simulink model "Lab5"  (R2018b)
settings: Solver=VariableStepAuto  StartTime=0.0  StopTime=0.7  RelTol=1e-3
values from neighbouring files (symbols this model uses):
  kpp = w_cp    (= 60)    [Lab5.m]
  kpv1 = w_cv/mu1    (= 0.09888)    [Lab5.m]
  kpv2 = w_cv/mu2    (= 0.114)    [Lab5.m]
  kpv3 = w_cv/mu3    (= 0.0408)    [Lab5.m]
  kpv4 = w_cv/mu4    (= 0.004056)    [Lab5.m]
  kpv5 = w_cv/mu5    (= 0.0031338)    [Lab5.m]
  kpv6 = w_cv/mu6    (= 0.003006)    [Lab5.m]
  n1 = 100    [Lab5.m]
  n2 = n1    (= 100)    [Lab5.m]
  n3 = n1    (= 100)    [Lab5.m]
  n4 = n1    (= 100)    [Lab5.m]
  n5 = n1    (= 100)    [Lab5.m]
  n6 = n1    (= 100)    [Lab5.m]
  t0 = 0.1    [Lab5.m]
  t_acc = (t_tot*x_dot_max-x_displacement)/x_dot_max    (= 0.1)    [Lab5.m]
  t_tot = 0.5    [Lab5.m]
  Tiv = 1/(0.2*w_cv)    (= 0.00833333333333)    [Lab5.m]
  x0 = 0.2    [Lab5.m]
  x_dotdot = x_dot_max/t_acc    (= 10)    [Lab5.m]
libraries: simulink x6, roblocks x1
settings Model: Creator=costanza  LastModifiedBy=costanza

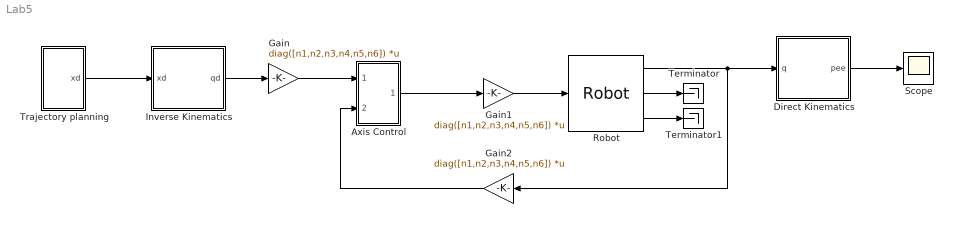
== system Lab5 ==
  "Axis Control " : Subsystem
  Direct Kinematics : Subsystem
  Gain : Gain  Gain=diag([n1,n2,n3,n4,n5,n6])  Multiplication=Matrix(K*u)
  Gain1 : Gain  Gain=diag([n1,n2,n3,n4,n5,n6])  Multiplication=Matrix(K*u)
  Gain2 : Gain  Gain=diag([n1,n2,n3,n4,n5,n6])  Multiplication=Matrix(K*u)
  Inverse Kinematics : Subsystem
  Robot : roblocks/Arm/Robot  robot=UR5  q0=q_init'
  Scope : Scope
  Terminator : Terminator
  Terminator1 : Terminator
  "Trajectory planning " : Subsystem
  wires:
  Gain/1 -> "Axis Control "/1(qmd)
  "Axis Control "/1("taum ") -> Gain1/1
  Gain1/1 -> Robot/1
  Robot/2 -> Terminator/1
  Robot/3 -> Terminator1/1
  Gain2/1 -> "Axis Control "/2(qm)
  Robot/1 -> Direct Kinematics/1("q "), Gain2/1
  Direct Kinematics/1(pee) -> Scope/1
  "Trajectory planning "/1(xd) -> Inverse Kinematics/1(xd)
  Inverse Kinematics/1(qd) -> Gain/1

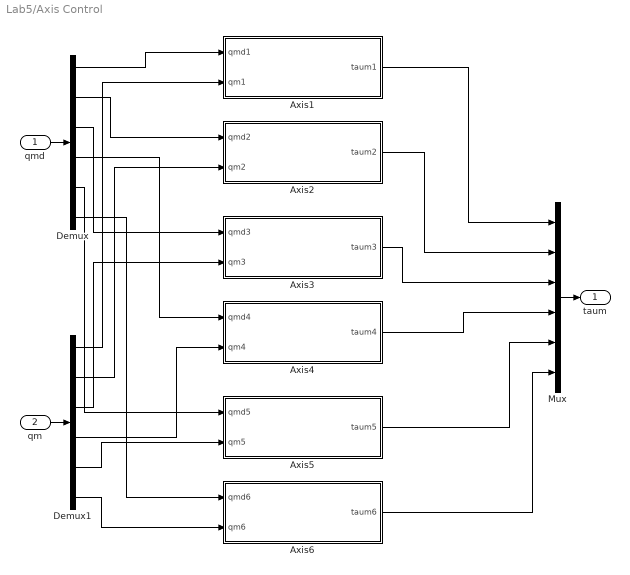
== system Lab5/Axis Control  ==
  qmd : Inport
  qm : Inport  Port=2
  "Axis1 " : Subsystem
  "Axis2 " : Subsystem
  "Axis3 " : Subsystem
  "Axis4 " : Subsystem
  "Axis5 " : Subsystem
  "Axis6 " : Subsystem
  Demux : Demux  Outputs=6
  Demux1 : Demux  Outputs=6
  Mux : Mux  Inputs=6
  "taum " : Outport
  wires:
  "Axis5 "/1(taum5) -> Mux/5
  Demux1/1 -> "Axis1 "/2(qm1)
  "Axis2 "/1(taum2) -> Mux/2
  Demux1/3 -> "Axis3 "/2(qm3)
  Demux/1 -> "Axis1 "/1(qmd1)
  "Axis4 "/1(taum4) -> Mux/4
  "Axis3 "/1(taum3) -> Mux/3
  "Axis6 "/1("taum6 ") -> Mux/6
  "Axis1 "/1(taum1) -> Mux/1
  Mux/1 -> "taum "/1
  Demux/2 -> "Axis2 "/1(qmd2)
  Demux/4 -> "Axis4 "/1(qmd4)
  Demux/3 -> "Axis3 "/1(qmd3)
  Demux/6 -> "Axis6 "/1(qmd6)
  Demux/5 -> "Axis5 "/1(qmd5)
  Demux1/4 -> "Axis4 "/2(qm4)
  Demux1/6 -> "Axis6 "/2(qm6)
  Demux1/5 -> "Axis5 "/2(qm5)
  Demux1/2 -> "Axis2 "/2(qm2)
  qm/1 -> Demux1/1
  qmd/1 -> Demux/1

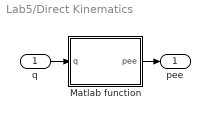
== system Lab5/Direct Kinematics ==
  "q " : Inport
  "Matlab function " : MATLAB Function  TreatAsAtomicUnit=on
  pee : Outport
  wires:
  "q "/1 -> "Matlab function "/1(q)
  "Matlab function "/1(pee) -> pee/1

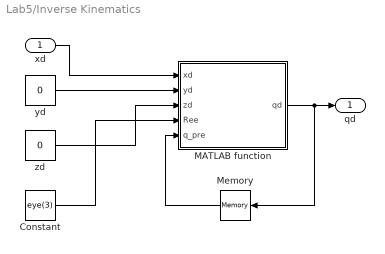
== system Lab5/Inverse Kinematics ==
  xd : Inport
  Constant : Constant  Value=eye(3)  VectorParams1D=off
  "MATLAB function " : MATLAB Function  TreatAsAtomicUnit=on
  Memory : Memory  InitialCondition=q_init'
  yd : Constant  Value=0
  "zd " : Constant  Value=0
  qd : Outport
  wires:
  xd/1 -> "MATLAB function "/1(xd)
  "MATLAB function "/1(qd) -> Memory/1, qd/1
  yd/1 -> "MATLAB function "/2(yd)
  "zd "/1 -> "MATLAB function "/3(zd)
  Constant/1 -> "MATLAB function "/4(Ree)
  Memory/1 -> "MATLAB function "/5(q_pre)

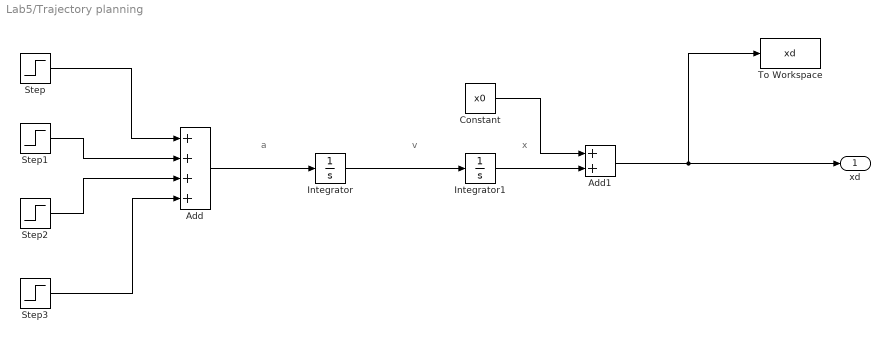
== system Lab5/Trajectory planning  ==
  note: a
  note: v
  note: x
  Add : Sum  Inputs=++++
  Add1 : Sum
  Constant : Constant  Value=x0
  Integrator : Integrator
  Integrator1 : Integrator
  Step : Step  Time=t0  After=x_dotdot  SampleTime=0
  Step1 : Step  Time=t0+t_acc  After=-x_dotdot  SampleTime=0
  Step2 : Step  Time=t0+t_tot-t_acc  After=-x_dotdot  SampleTime=0
  Step3 : Step  Time=t0+t_tot  After=x_dotdot  SampleTime=0
  To Workspace : ToWorkspace  VariableName=xd  SampleTime=-1
  xd : Outport
  wires:
  Step2/1 -> Add/3
  Step/1 -> Add/1
  Add/1 -> Integrator/1
  Step3/1 -> Add/4
  Step1/1 -> Add/2
  Integrator/1 -> Integrator1/1
  Add1/1 -> xd/1, To Workspace/1
  Constant/1 -> Add1/1
  Integrator1/1 -> Add1/2

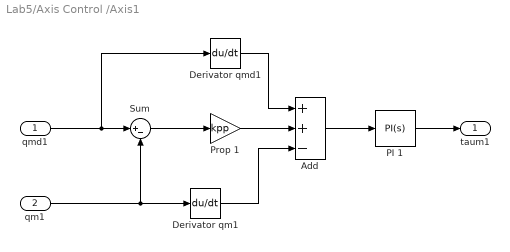
== system Lab5/Axis Control /Axis1  ==
  qmd1 : Inport
  qm1 : Inport  Port=2
  Add : Sum  Inputs=++-
  Derivator qm1 : Derivative  CoefficientInTFapproximation=1/260
  "Derivator qmd1 " : Derivative  CoefficientInTFapproximation=1/260
  PI 1 : simulink/Continuous/PID Controller  Controller=PI  Form=Parallel  TimeDomain=Continuous-time  SampleTime=-1  IntegratorMethod=Forward Euler  FilterMethod=Forward Euler  ControllerParametersSource=internal  P=kpv1  I=kpv1/Tiv  D=0  UseFilter=on  N=100  TunerSelectOption=Transfer Function Based (PID Tuner App)  InitialConditionSource=internal  InitialConditionForIntegrator=0  InitialConditionForFilter=0  DifferentiatorICPrevScaledInput=0  ExternalReset=none  TrackingMode=off  Kt=1  LimitOutput=off  UpperSaturationLimit=inf  LowerSaturationLimit=-inf  LinearizeAsGain=on  AntiWindupMode=none  Kb=1  POutMin=[]  POutMax=[]  IOutMin=[]  IOutMax=[]  DOutMin=[]  DOutMax=[]  NOutMin=[]  NOutMax=[]  SumOutMin=[]  SumOutMax=[]  SaturationOutMin=[]  SaturationOutMax=[]  PParamMin=[]  PParamMax=[]  IParamMin=[]  IParamMax=[]  DParamMin=[]  DParamMax=[]  NParamMin=[]  NParamMax=[]  KbParamMin=[]  KbParamMax=[]  KtParamMin=[]  KtParamMax=[]  KbOutMin=[]  KbOutMax=[]  KtOutMin=[]  KtOutMax=[]  IntegratorOutMin=[]  IntegratorOutMax=[]  FilterOutMin=[]  FilterOutMax=[]  SumI1OutMin=[]  SumI1OutMax=[]  SumI2OutMin=[]  SumI2OutMax=[]  SumI3OutMin=[]  SumI3OutMax=[]  SumI4OutMin=[]  SumI4OutMax=[]  SumDOutMin=[]  SumDOutMax=[]  DifferentiatorOutMin=[]  DifferentiatorOutMax=[]  FilterDiffOutCoefMin=[]  FilterDiffOutCoefMax=[]  ReciprocalOutMin=[]  ReciprocalOutMax=[]  SumDenOutMin=[]  SumDenOutMax=[]  SumNumOutMin=[]  SumNumOutMax=[]  DivideOutMin=[]  DivideOutMax=[]  IntegratorContinuousStateAttributes=''  IntegratorStateMustResolveToSignalObject=off  IntegratorRTWStateStorageClass=Auto  FilterContinuousStateAttributes=''  FilterStateMustResolveToSignalObject=off  FilterRTWStateStorageClass=Auto  ParallelPVariant=InternalParameters  IdealPVariant=Disabled  IVariant=InternalParameters  DVariant=Disabled  IntegratorVariant=Continuous  SatVariant=Disabled  AWVariant=Passthrough  PCopyVariant=Disabled  TRVariant=Disabled  FdbkBlocksVariant=Forward  IdealPFdbkVariant=Disabled  SatFdbkVariant=Disabled  DerivativeFilterVariant=Disabled  NVariant=Disabled  NCopyVariant=Disabled_SignalSpec  FilterICVariant=Disabled  IntegratorICVariant=InternalICs  ExternalResetVariant=Disabled  TRSumVariant=Passthrough  SumFdbkVariant=Disabled  SumVariant=Sum_PI
  Prop 1 : Gain  Gain=kpp
  Sum : Sum  Inputs=|+-
  taum1 : Outport
  wires:
  "Derivator qmd1 "/1 -> Add/1
  Derivator qm1/1 -> Add/3
  Sum/1 -> Prop 1/1
  qm1/1 -> Derivator qm1/1, Sum/2
  Prop 1/1 -> Add/2
  Add/1 -> PI 1/1
  qmd1/1 -> "Derivator qmd1 "/1, Sum/1
  PI 1/1 -> taum1/1

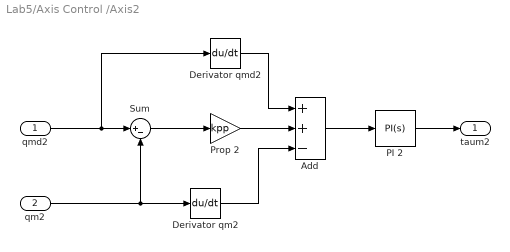
== system Lab5/Axis Control /Axis2  ==
  qmd2 : Inport
  qm2 : Inport  Port=2
  Add : Sum  Inputs=++-
  Derivator qm2 : Derivative  CoefficientInTFapproximation=1/260
  Derivator qmd2 : Derivative  CoefficientInTFapproximation=1/260
  PI 2 : simulink/Continuous/PID Controller  Controller=PI  Form=Parallel  TimeDomain=Continuous-time  SampleTime=-1  IntegratorMethod=Forward Euler  FilterMethod=Forward Euler  ControllerParametersSource=internal  P=kpv2  I=kpv2/Tiv  D=0  UseFilter=on  N=100  TunerSelectOption=Transfer Function Based (PID Tuner App)  InitialConditionSource=internal  InitialConditionForIntegrator=0  InitialConditionForFilter=0  DifferentiatorICPrevScaledInput=0  ExternalReset=none  TrackingMode=off  Kt=1  LimitOutput=off  UpperSaturationLimit=inf  LowerSaturationLimit=-inf  LinearizeAsGain=on  AntiWindupMode=none  Kb=1  POutMin=[]  POutMax=[]  IOutMin=[]  IOutMax=[]  DOutMin=[]  DOutMax=[]  NOutMin=[]  NOutMax=[]  SumOutMin=[]  SumOutMax=[]  SaturationOutMin=[]  SaturationOutMax=[]  PParamMin=[]  PParamMax=[]  IParamMin=[]  IParamMax=[]  DParamMin=[]  DParamMax=[]  NParamMin=[]  NParamMax=[]  KbParamMin=[]  KbParamMax=[]  KtParamMin=[]  KtParamMax=[]  KbOutMin=[]  KbOutMax=[]  KtOutMin=[]  KtOutMax=[]  IntegratorOutMin=[]  IntegratorOutMax=[]  FilterOutMin=[]  FilterOutMax=[]  SumI1OutMin=[]  SumI1OutMax=[]  SumI2OutMin=[]  SumI2OutMax=[]  SumI3OutMin=[]  SumI3OutMax=[]  SumI4OutMin=[]  SumI4OutMax=[]  SumDOutMin=[]  SumDOutMax=[]  DifferentiatorOutMin=[]  DifferentiatorOutMax=[]  FilterDiffOutCoefMin=[]  FilterDiffOutCoefMax=[]  ReciprocalOutMin=[]  ReciprocalOutMax=[]  SumDenOutMin=[]  SumDenOutMax=[]  SumNumOutMin=[]  SumNumOutMax=[]  DivideOutMin=[]  DivideOutMax=[]  IntegratorContinuousStateAttributes=''  IntegratorStateMustResolveToSignalObject=off  IntegratorRTWStateStorageClass=Auto  FilterContinuousStateAttributes=''  FilterStateMustResolveToSignalObject=off  FilterRTWStateStorageClass=Auto  ParallelPVariant=InternalParameters  IdealPVariant=Disabled  IVariant=InternalParameters  DVariant=Disabled  IntegratorVariant=Continuous  SatVariant=Disabled  AWVariant=Passthrough  PCopyVariant=Disabled  TRVariant=Disabled  FdbkBlocksVariant=Forward  IdealPFdbkVariant=Disabled  SatFdbkVariant=Disabled  DerivativeFilterVariant=Disabled  NVariant=Disabled  NCopyVariant=Disabled_SignalSpec  FilterICVariant=Disabled  IntegratorICVariant=InternalICs  ExternalResetVariant=Disabled  TRSumVariant=Passthrough  SumFdbkVariant=Disabled  SumVariant=Sum_PI
  Prop 2 : Gain  Gain=kpp
  Sum : Sum  Inputs=|+-
  taum2 : Outport
  wires:
  Derivator qmd2/1 -> Add/1
  Derivator qm2/1 -> Add/3
  Sum/1 -> Prop 2/1
  qm2/1 -> Derivator qm2/1, Sum/2
  Prop 2/1 -> Add/2
  Add/1 -> PI 2/1
  qmd2/1 -> Derivator qmd2/1, Sum/1
  PI 2/1 -> taum2/1

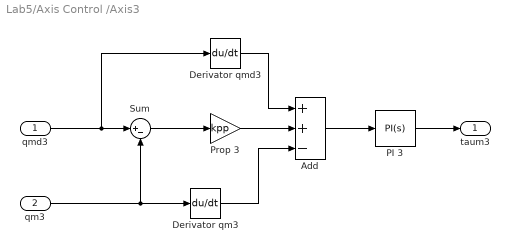
== system Lab5/Axis Control /Axis3  ==
  qmd3 : Inport
  qm3 : Inport  Port=2
  Add : Sum  Inputs=++-
  Derivator qm3 : Derivative  CoefficientInTFapproximation=1/260
  Derivator qmd3 : Derivative  CoefficientInTFapproximation=1/260
  PI 3 : simulink/Continuous/PID Controller  Controller=PI  Form=Parallel  TimeDomain=Continuous-time  SampleTime=-1  IntegratorMethod=Forward Euler  FilterMethod=Forward Euler  ControllerParametersSource=internal  P=kpv3  I=kpv3/Tiv  D=0  UseFilter=on  N=100  TunerSelectOption=Transfer Function Based (PID Tuner App)  InitialConditionSource=internal  InitialConditionForIntegrator=0  InitialConditionForFilter=0  DifferentiatorICPrevScaledInput=0  ExternalReset=none  TrackingMode=off  Kt=1  LimitOutput=off  UpperSaturationLimit=inf  LowerSaturationLimit=-inf  LinearizeAsGain=on  AntiWindupMode=none  Kb=1  POutMin=[]  POutMax=[]  IOutMin=[]  IOutMax=[]  DOutMin=[]  DOutMax=[]  NOutMin=[]  NOutMax=[]  SumOutMin=[]  SumOutMax=[]  SaturationOutMin=[]  SaturationOutMax=[]  PParamMin=[]  PParamMax=[]  IParamMin=[]  IParamMax=[]  DParamMin=[]  DParamMax=[]  NParamMin=[]  NParamMax=[]  KbParamMin=[]  KbParamMax=[]  KtParamMin=[]  KtParamMax=[]  KbOutMin=[]  KbOutMax=[]  KtOutMin=[]  KtOutMax=[]  IntegratorOutMin=[]  IntegratorOutMax=[]  FilterOutMin=[]  FilterOutMax=[]  SumI1OutMin=[]  SumI1OutMax=[]  SumI2OutMin=[]  SumI2OutMax=[]  SumI3OutMin=[]  SumI3OutMax=[]  SumI4OutMin=[]  SumI4OutMax=[]  SumDOutMin=[]  SumDOutMax=[]  DifferentiatorOutMin=[]  DifferentiatorOutMax=[]  FilterDiffOutCoefMin=[]  FilterDiffOutCoefMax=[]  ReciprocalOutMin=[]  ReciprocalOutMax=[]  SumDenOutMin=[]  SumDenOutMax=[]  SumNumOutMin=[]  SumNumOutMax=[]  DivideOutMin=[]  DivideOutMax=[]  IntegratorContinuousStateAttributes=''  IntegratorStateMustResolveToSignalObject=off  IntegratorRTWStateStorageClass=Auto  FilterContinuousStateAttributes=''  FilterStateMustResolveToSignalObject=off  FilterRTWStateStorageClass=Auto  ParallelPVariant=InternalParameters  IdealPVariant=Disabled  IVariant=InternalParameters  DVariant=Disabled  IntegratorVariant=Continuous  SatVariant=Disabled  AWVariant=Passthrough  PCopyVariant=Disabled  TRVariant=Disabled  FdbkBlocksVariant=Forward  IdealPFdbkVariant=Disabled  SatFdbkVariant=Disabled  DerivativeFilterVariant=Disabled  NVariant=Disabled  NCopyVariant=Disabled_SignalSpec  FilterICVariant=Disabled  IntegratorICVariant=InternalICs  ExternalResetVariant=Disabled  TRSumVariant=Passthrough  SumFdbkVariant=Disabled  SumVariant=Sum_PI
  Prop 3 : Gain  Gain=kpp
  Sum : Sum  Inputs=|+-
  taum3 : Outport
  wires:
  Derivator qmd3/1 -> Add/1
  Derivator qm3/1 -> Add/3
  Sum/1 -> Prop 3/1
  qm3/1 -> Derivator qm3/1, Sum/2
  Prop 3/1 -> Add/2
  Add/1 -> PI 3/1
  qmd3/1 -> Derivator qmd3/1, Sum/1
  PI 3/1 -> taum3/1

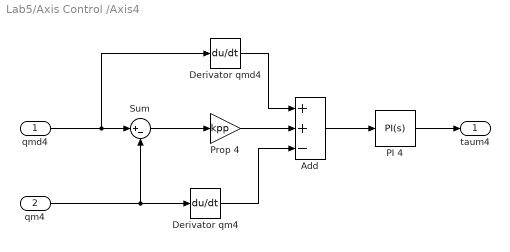
== system Lab5/Axis Control /Axis4  ==
  qmd4 : Inport
  qm4 : Inport  Port=2
  Add : Sum  Inputs=++-
  Derivator qm4 : Derivative  CoefficientInTFapproximation=1/700
  Derivator qmd4 : Derivative  CoefficientInTFapproximation=1/700
  PI 4 : simulink/Continuous/PID Controller  Controller=PI  Form=Parallel  TimeDomain=Continuous-time  SampleTime=-1  IntegratorMethod=Forward Euler  FilterMethod=Forward Euler  ControllerParametersSource=internal  P=kpv4  I=kpv4/Tiv  D=0  UseFilter=on  N=100  TunerSelectOption=Transfer Function Based (PID Tuner App)  InitialConditionSource=internal  InitialConditionForIntegrator=0  InitialConditionForFilter=0  DifferentiatorICPrevScaledInput=0  ExternalReset=none  TrackingMode=off  Kt=1  LimitOutput=off  UpperSaturationLimit=inf  LowerSaturationLimit=-inf  LinearizeAsGain=on  AntiWindupMode=none  Kb=1  POutMin=[]  POutMax=[]  IOutMin=[]  IOutMax=[]  DOutMin=[]  DOutMax=[]  NOutMin=[]  NOutMax=[]  SumOutMin=[]  SumOutMax=[]  SaturationOutMin=[]  SaturationOutMax=[]  PParamMin=[]  PParamMax=[]  IParamMin=[]  IParamMax=[]  DParamMin=[]  DParamMax=[]  NParamMin=[]  NParamMax=[]  KbParamMin=[]  KbParamMax=[]  KtParamMin=[]  KtParamMax=[]  KbOutMin=[]  KbOutMax=[]  KtOutMin=[]  KtOutMax=[]  IntegratorOutMin=[]  IntegratorOutMax=[]  FilterOutMin=[]  FilterOutMax=[]  SumI1OutMin=[]  SumI1OutMax=[]  SumI2OutMin=[]  SumI2OutMax=[]  SumI3OutMin=[]  SumI3OutMax=[]  SumI4OutMin=[]  SumI4OutMax=[]  SumDOutMin=[]  SumDOutMax=[]  DifferentiatorOutMin=[]  DifferentiatorOutMax=[]  FilterDiffOutCoefMin=[]  FilterDiffOutCoefMax=[]  ReciprocalOutMin=[]  ReciprocalOutMax=[]  SumDenOutMin=[]  SumDenOutMax=[]  SumNumOutMin=[]  SumNumOutMax=[]  DivideOutMin=[]  DivideOutMax=[]  IntegratorContinuousStateAttributes=''  IntegratorStateMustResolveToSignalObject=off  IntegratorRTWStateStorageClass=Auto  FilterContinuousStateAttributes=''  FilterStateMustResolveToSignalObject=off  FilterRTWStateStorageClass=Auto  ParallelPVariant=InternalParameters  IdealPVariant=Disabled  IVariant=InternalParameters  DVariant=Disabled  IntegratorVariant=Continuous  SatVariant=Disabled  AWVariant=Passthrough  PCopyVariant=Disabled  TRVariant=Disabled  FdbkBlocksVariant=Forward  IdealPFdbkVariant=Disabled  SatFdbkVariant=Disabled  DerivativeFilterVariant=Disabled  NVariant=Disabled  NCopyVariant=Disabled_SignalSpec  FilterICVariant=Disabled  IntegratorICVariant=InternalICs  ExternalResetVariant=Disabled  TRSumVariant=Passthrough  SumFdbkVariant=Disabled  SumVariant=Sum_PI
  Prop 4 : Gain  Gain=kpp
  Sum : Sum  Inputs=|+-
  taum4 : Outport
  wires:
  Derivator qmd4/1 -> Add/1
  Derivator qm4/1 -> Add/3
  Sum/1 -> Prop 4/1
  qm4/1 -> Derivator qm4/1, Sum/2
  Prop 4/1 -> Add/2
  Add/1 -> PI 4/1
  qmd4/1 -> Derivator qmd4/1, Sum/1
  PI 4/1 -> taum4/1

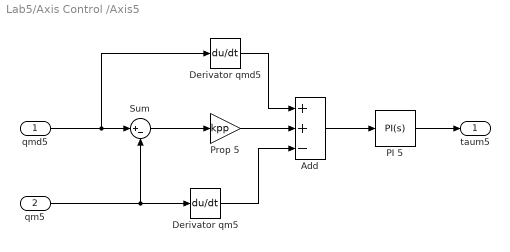
== system Lab5/Axis Control /Axis5  ==
  qmd5 : Inport
  qm5 : Inport  Port=2
  Add : Sum  Inputs=++-
  Derivator qm5 : Derivative  CoefficientInTFapproximation=1/700
  Derivator qmd5 : Derivative  CoefficientInTFapproximation=1/700
  PI 5 : simulink/Continuous/PID Controller  Controller=PI  Form=Parallel  TimeDomain=Continuous-time  SampleTime=-1  IntegratorMethod=Forward Euler  FilterMethod=Forward Euler  ControllerParametersSource=internal  P=kpv5  I=kpv5/Tiv  D=0  UseFilter=on  N=100  TunerSelectOption=Transfer Function Based (PID Tuner App)  InitialConditionSource=internal  InitialConditionForIntegrator=0  InitialConditionForFilter=0  DifferentiatorICPrevScaledInput=0  ExternalReset=none  TrackingMode=off  Kt=1  LimitOutput=off  UpperSaturationLimit=inf  LowerSaturationLimit=-inf  LinearizeAsGain=on  AntiWindupMode=none  Kb=1  POutMin=[]  POutMax=[]  IOutMin=[]  IOutMax=[]  DOutMin=[]  DOutMax=[]  NOutMin=[]  NOutMax=[]  SumOutMin=[]  SumOutMax=[]  SaturationOutMin=[]  SaturationOutMax=[]  PParamMin=[]  PParamMax=[]  IParamMin=[]  IParamMax=[]  DParamMin=[]  DParamMax=[]  NParamMin=[]  NParamMax=[]  KbParamMin=[]  KbParamMax=[]  KtParamMin=[]  KtParamMax=[]  KbOutMin=[]  KbOutMax=[]  KtOutMin=[]  KtOutMax=[]  IntegratorOutMin=[]  IntegratorOutMax=[]  FilterOutMin=[]  FilterOutMax=[]  SumI1OutMin=[]  SumI1OutMax=[]  SumI2OutMin=[]  SumI2OutMax=[]  SumI3OutMin=[]  SumI3OutMax=[]  SumI4OutMin=[]  SumI4OutMax=[]  SumDOutMin=[]  SumDOutMax=[]  DifferentiatorOutMin=[]  DifferentiatorOutMax=[]  FilterDiffOutCoefMin=[]  FilterDiffOutCoefMax=[]  ReciprocalOutMin=[]  ReciprocalOutMax=[]  SumDenOutMin=[]  SumDenOutMax=[]  SumNumOutMin=[]  SumNumOutMax=[]  DivideOutMin=[]  DivideOutMax=[]  IntegratorContinuousStateAttributes=''  IntegratorStateMustResolveToSignalObject=off  IntegratorRTWStateStorageClass=Auto  FilterContinuousStateAttributes=''  FilterStateMustResolveToSignalObject=off  FilterRTWStateStorageClass=Auto  ParallelPVariant=InternalParameters  IdealPVariant=Disabled  IVariant=InternalParameters  DVariant=Disabled  IntegratorVariant=Continuous  SatVariant=Disabled  AWVariant=Passthrough  PCopyVariant=Disabled  TRVariant=Disabled  FdbkBlocksVariant=Forward  IdealPFdbkVariant=Disabled  SatFdbkVariant=Disabled  DerivativeFilterVariant=Disabled  NVariant=Disabled  NCopyVariant=Disabled_SignalSpec  FilterICVariant=Disabled  IntegratorICVariant=InternalICs  ExternalResetVariant=Disabled  TRSumVariant=Passthrough  SumFdbkVariant=Disabled  SumVariant=Sum_PI
  Prop 5 : Gain  Gain=kpp
  Sum : Sum  Inputs=|+-
  taum5 : Outport
  wires:
  Derivator qmd5/1 -> Add/1
  Derivator qm5/1 -> Add/3
  Sum/1 -> Prop 5/1
  qm5/1 -> Derivator qm5/1, Sum/2
  Prop 5/1 -> Add/2
  Add/1 -> PI 5/1
  qmd5/1 -> Derivator qmd5/1, Sum/1
  PI 5/1 -> taum5/1

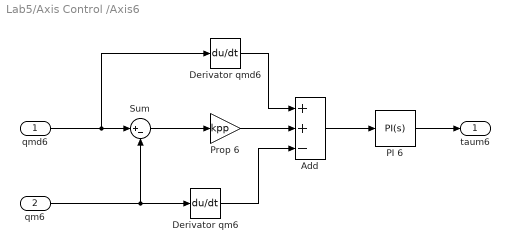
== system Lab5/Axis Control /Axis6  ==
  qmd6 : Inport
  qm6 : Inport  Port=2
  Add : Sum  Inputs=++-
  Derivator qm6 : Derivative  CoefficientInTFapproximation=1/700
  Derivator qmd6 : Derivative  CoefficientInTFapproximation=1/700
  PI 6 : simulink/Continuous/PID Controller  Controller=PI  Form=Parallel  TimeDomain=Continuous-time  SampleTime=-1  IntegratorMethod=Forward Euler  FilterMethod=Forward Euler  ControllerParametersSource=internal  P=kpv6  I=kpv6/Tiv  D=0  UseFilter=on  N=100  TunerSelectOption=Transfer Function Based (PID Tuner App)  InitialConditionSource=internal  InitialConditionForIntegrator=0  InitialConditionForFilter=0  DifferentiatorICPrevScaledInput=0  ExternalReset=none  TrackingMode=off  Kt=1  LimitOutput=off  UpperSaturationLimit=inf  LowerSaturationLimit=-inf  LinearizeAsGain=on  AntiWindupMode=none  Kb=1  POutMin=[]  POutMax=[]  IOutMin=[]  IOutMax=[]  DOutMin=[]  DOutMax=[]  NOutMin=[]  NOutMax=[]  SumOutMin=[]  SumOutMax=[]  SaturationOutMin=[]  SaturationOutMax=[]  PParamMin=[]  PParamMax=[]  IParamMin=[]  IParamMax=[]  DParamMin=[]  DParamMax=[]  NParamMin=[]  NParamMax=[]  KbParamMin=[]  KbParamMax=[]  KtParamMin=[]  KtParamMax=[]  KbOutMin=[]  KbOutMax=[]  KtOutMin=[]  KtOutMax=[]  IntegratorOutMin=[]  IntegratorOutMax=[]  FilterOutMin=[]  FilterOutMax=[]  SumI1OutMin=[]  SumI1OutMax=[]  SumI2OutMin=[]  SumI2OutMax=[]  SumI3OutMin=[]  SumI3OutMax=[]  SumI4OutMin=[]  SumI4OutMax=[]  SumDOutMin=[]  SumDOutMax=[]  DifferentiatorOutMin=[]  DifferentiatorOutMax=[]  FilterDiffOutCoefMin=[]  FilterDiffOutCoefMax=[]  ReciprocalOutMin=[]  ReciprocalOutMax=[]  SumDenOutMin=[]  SumDenOutMax=[]  SumNumOutMin=[]  SumNumOutMax=[]  DivideOutMin=[]  DivideOutMax=[]  IntegratorContinuousStateAttributes=''  IntegratorStateMustResolveToSignalObject=off  IntegratorRTWStateStorageClass=Auto  FilterContinuousStateAttributes=''  FilterStateMustResolveToSignalObject=off  FilterRTWStateStorageClass=Auto  ParallelPVariant=InternalParameters  IdealPVariant=Disabled  IVariant=InternalParameters  DVariant=Disabled  IntegratorVariant=Continuous  SatVariant=Disabled  AWVariant=Passthrough  PCopyVariant=Disabled  TRVariant=Disabled  FdbkBlocksVariant=Forward  IdealPFdbkVariant=Disabled  SatFdbkVariant=Disabled  DerivativeFilterVariant=Disabled  NVariant=Disabled  NCopyVariant=Disabled_SignalSpec  FilterICVariant=Disabled  IntegratorICVariant=InternalICs  ExternalResetVariant=Disabled  TRSumVariant=Passthrough  SumFdbkVariant=Disabled  SumVariant=Sum_PI
  Prop 6 : Gain  Gain=kpp
  Sum : Sum  Inputs=|+-
  "taum6 " : Outport
  wires:
  Derivator qmd6/1 -> Add/1
  Derivator qm6/1 -> Add/3
  Sum/1 -> Prop 6/1
  qm6/1 -> Derivator qm6/1, Sum/2
  Prop 6/1 -> Add/2
  Add/1 -> PI 6/1
  qmd6/1 -> Derivator qmd6/1, Sum/1
  PI 6/1 -> "taum6 "/1

== matlab function Lab5/Direct Kinematics/Matlab function  ==
  data: q input; pee output
function pee = ComputeDK(q)
%#codegen
u1=q(1);
u2=q(2);
u3=q(3);
u4=q(4);
u5=q(5);
u6=q(6);
%DH param
alpha = [pi/2,0,0,pi/2,-pi/2,0]; %[in rad]
a = [0,-0.425,-0.39225,0,0,0]; %[in m]
d = [0.08916,0,0,0.10915,0.09456,0.0823]; %[in m]

A10=[cos(u1) -sin(u1)*cos(alpha(1,1)) sin(u1)*sin(alpha(1,1)) a(1,1)*cos(u1);
    sin(u1) cos(u1)*cos(alpha(1,1)) -cos(u1)*sin(alpha(1,1)) a(1,1)*sin(u1);
    0 sin(alpha(1,1)) cos(alpha(1,1)) d(1,1);
    0 0 0 1];
A21=[cos(u2) -sin(u2)*cos(alpha(1,2)) sin(u2)*sin(alpha(1,2)) a(1,2)*cos(u2);
    sin(u2) cos(u2)*cos(alpha(1,2)) -cos(u2)*sin(alpha(1,2)) a(1,2)*sin(u2);
    0 sin(alpha(1,2)) cos(alpha(1,2)) d(1,2);
    0 0 0 1];
A32=[cos(u3) -sin(u3)*cos(alpha(1,3)) sin(u3)*sin(alpha(1,3)) a(1,3)*cos(u3);
    sin(u3) cos(u3)*cos(alpha(1,3)) -cos(u3)*sin(alpha(1,3)) a(1,3)*sin(u3);
    0 sin(alpha(1,3)) cos(alpha(1,3)) d(1,3);
    0 0 0 1];
A43=[cos(u4) -sin(u4)*cos(alpha(1,4)) sin(u4)*sin(alpha(1,4)) a(1,4)*cos(u4);
    sin(u4) cos(u4)*cos(alpha(1,4)) -cos(u4)*sin(alpha(1,4)) a(1,4)*sin(u4);
    0 sin(alpha(1,4)) cos(alpha(1,4)) d(1,4);
    0 0 0 1];
A54=[cos(u5) -sin(u5)*cos(alpha(1,5)) sin(u5)*sin(alpha(1,5)) a(1,5)*cos(u5);
    sin(u5) cos(u5)*cos(alpha(1,5)) -cos(u5)*sin(alpha(1,5)) a(1,5)*sin(u5);
    0 sin(alpha(1,5)) cos(alpha(1,5)) d(1,5);
    0 0 0 1];
A65=[cos(u6) -sin(u6)*cos(alpha(1,6)) sin(u6)*sin(alpha(1,6)) a(1,6)*cos(u6);
    sin(u6) cos(u6)*cos(alpha(1,6)) -cos(u6)*sin(alpha(1,6)) a(1,6)*sin(u6);
    0 sin(alpha(1,6)) cos(alpha(1,6)) d(1,6);
    0 0 0 1];
A60=A10*A21*A32*A43*A54*A65;
pee = A60(1:3,4); %x,y,z

== matlab function Lab5/Inverse Kinematics/MATLAB function  ==
  data: xd input; qd output; yd input; zd input; Ree input; q_pre input
function qd = ComputeIK(xd,yd,zd,Ree,q_pre)
%q_pre is a column vector
%DH param
alpha = [pi/2,0,0,pi/2,-pi/2,0]; %[in rad]
a = [0,-0.425,-0.39225,0,0,0]; %[in m]
d = [0.08916,0,0,0.10915,0.09465,0.0823]; %[in m]

ee_pos_desired = [xd yd zd]; %desired position of the end effector
T60=[Ree ee_pos_desired';
    zeros(1,3) 1];
p50=T60*[0 0 -d(1,6) 1]'-[0 0 0 1]';
psi=atan2(p50(2,1),p50(1,1));
argacosphi=d(1,4)/(sqrt(p50(1,1)^2+p50(2,1)^2));
phi1=acos(max(min(argacosphi,1),-1)); %bound acos argument between -1 and 1
phi2=-acos(max(min(argacosphi,1),-1)); %bound acos argument between -1 and 1
Theta_11=psi+phi1+pi/2; %shoulder left
Theta_12=psi+phi2+pi/2; %shoulder right

p60=ee_pos_desired';
p61_z1=p60(1,1)*sin(Theta_11)-p60(2,1)*cos(Theta_11);
p61_z2=p60(1,1)*sin(Theta_12)-p60(2,1)*cos(Theta_12);
argacos51=(p61_z1-d(1,4))/d(1,6); %bound acos argument between -1 and 1
argacos52=(p61_z2-d(1,4))/d(1,6); %bound acos argument between -1 and 1
Theta_51=acos(max(min(argacos51,1),-1));
Theta_52=-acos(max(min(argacos51,1),-1));
Theta_53=acos(max(min(argacos52,1),-1));
Theta_54=-acos(max(min(argacos52,1),-1));

T10_1=[cos(Theta_11) -sin(Theta_11)*cos(alpha(1,1)) sin(Theta_11)*sin(alpha(1,1)) a(1,1)*cos(Theta_11);
    sin(Theta_11) cos(Theta_11)*cos(alpha(1,1)) -cos(Theta_11)*sin(alpha(1,1)) a(1,1)*sin(Theta_11);
    0 sin(alpha(1,1)) cos(alpha(1,1)) d(1,1);
    0 0 0 1];
T10_2=[cos(Theta_12) -sin(Theta_12)*cos(alpha(1,1)) sin(Theta_12)*sin(alpha(1,1)) a(1,1)*cos(Theta_12);
    sin(Theta_12) cos(Theta_12)*cos(alpha(1,1)) -cos(Theta_12)*sin(alpha(1,1)) a(1,1)*sin(Theta_12);
    0 sin(alpha(1,1)) cos(alpha(1,1)) d(1,1);
    0 0 0 1];

T16_1=inv(T60)*T10_1;
T16_2=inv(T60)*T10_2;
zy_1=T16_1(2,3);
zx_1=T16_1(1,3);
zy_2=T16_2(2,3);
zx_2=T16_2(1,3);
Theta_61=atan2(-zy_1/sin(Theta_51),zx_1/sin(Theta_51));
Theta_62=atan2(-zy_1/sin(Theta_52),zx_1/sin(Theta_52));
Theta_63=atan2(-zy_2/sin(Theta_53),zx_2/sin(Theta_53));
Theta_64=atan2(-zy_2/sin(Theta_54),zx_2/sin(Theta_54));


T61_1=inv(T16_1);
T61_2=inv(T16_2);
T54_1=[cos(Theta_51) -sin(Theta_51)*cos(alpha(1,5)) sin(Theta_51)*sin(alpha(1,5)) a(1,5)*cos(Theta_51);
    sin(Theta_51) cos(Theta_51)*cos(alpha(1,5)) -cos(Theta_51)*sin(alpha(1,5)) a(1,5)*sin(Theta_51);
    0 sin(alpha(1,5)) cos(alpha(1,5)) d(1,5);
    0 0 0 1];
T54_2=[cos(Theta_52) -sin(Theta_52)*cos(alpha(1,5)) sin(Theta_52)*sin(alpha(1,5)) a(1,5)*cos(Theta_52);
    sin(Theta_52) cos(Theta_52)*cos(alpha(1,5)) -cos(Theta_52)*sin(alpha(1,5)) a(1,5)*sin(Theta_52);
    0 sin(alpha(1,5)) cos(alpha(1,5)) d(1,5);
    0 0 0 1];
T54_3=[cos(Theta_53) -sin(Theta_53)*cos(alpha(1,5)) sin(Theta_53)*sin(alpha(1,5)) a(1,5)*cos(Theta_53);
    sin(Theta_53) cos(Theta_53)*cos(alpha(1,5)) -cos(Theta_53)*sin(alpha(1,5)) a(1,5)*sin(Theta_53);
    0 sin(alpha(1,5)) cos(alpha(1,5)) d(1,5);
    0 0 0 1];
T54_4=[cos(Theta_54) -sin(Theta_54)*cos(alpha(1,5)) sin(Theta_54)*sin(alpha(1,5)) a(1,5)*cos(Theta_54);
    sin(Theta_54) cos(Theta_54)*cos(alpha(1,5)) -cos(Theta_54)*sin(alpha(1,5)) a(1,5)*sin(Theta_54);
    0 sin(alpha(1,5)) cos(alpha(1,5)) d(1,5);
    0 0 0 1];

T65_1=[cos(Theta_61) -sin(Theta_61)*cos(alpha(1,6)) sin(Theta_61)*sin(alpha(1,6)) a(1,6)*cos(Theta_61);
    sin(Theta_61) cos(Theta_61)*cos(alpha(1,6)) -cos(Theta_61)*sin(alpha(1,6)) a(1,6)*sin(Theta_61);
    0 sin(alpha(1,6)) cos(alpha(1,6)) d(1,6);
    0 0 0 1];
T65_2=[cos(Theta_62) -sin(Theta_62)*cos(alpha(1,6)) sin(Theta_62)*sin(alpha(1,6)) a(1,6)*cos(Theta_62);
    sin(Theta_62) cos(Theta_62)*cos(alpha(1,6)) -cos(Theta_62)*sin(alpha(1,6)) a(1,6)*sin(Theta_62);
    0 sin(alpha(1,6)) cos(alpha(1,6)) d(1,6);
    0 0 0 1];
T65_3=[cos(Theta_63) -sin(Theta_63)*cos(alpha(1,6)) sin(Theta_63)*sin(alpha(1,6)) a(1,6)*cos(Theta_63);
    sin(Theta_63) cos(Theta_63)*cos(alpha(1,6)) -cos(Theta_63)*sin(alpha(1,6)) a(1,6)*sin(Theta_63);
    0 sin(alpha(1,6)) cos(alpha(1,6)) d(1,6);
    0 0 0 1];
T65_4=[cos(Theta_64) -sin(Theta_64)*cos(alpha(1,6)) sin(Theta_64)*sin(alpha(1,6)) a(1,6)*cos(Theta_64);
    sin(Theta_64) cos(Theta_64)*cos(alpha(1,6)) -cos(Theta_64)*sin(alpha(1,6)) a(1,6)*sin(Theta_64);
    0 sin(alpha(1,6)) cos(alpha(1,6)) d(1,6);
    0 0 0 1];



T41_1=T61_1/(T54_1*T65_1); %=T61*inv(T54*T65)
T41_2=T61_1/(T54_2*T65_2); %=T61*inv(T54*T65)
T41_3=T61_2/(T54_3*T65_3); %=T61*inv(T54*T65)
T41_4=T61_2/(T54_4*T65_4); %=T61*inv(T54*T65)


p31_1=T41_1*[0 -d(1,4) 0 1]'-[0 0 0 1]';
p31_2=T41_2*[0 -d(1,4) 0 1]'-[0 0 0 1]';
p31_3=T41_3*[0 -d(1,4) 0 1]'-[0 0 0 1]';
p31_4=T41_4*[0 -d(1,4) 0 1]'-[0 0 0 1]';

norm_p31_1=norm(p31_1);
norm_p31_2=norm(p31_2);
norm_p31_3=norm(p31_3);
norm_p31_4=norm(p31_4);

argacos3_1=(norm_p31_1^2-a(1,2)^2-a(1,3)^2)/(2*a(1,2)*a(1,3)); %bound acos argument between -1 and 1
argacos3_2=(norm_p31_2^2-a(1,2)^2-a(1,3)^2)/(2*a(1,2)*a(1,3)); %bound acos argument between -1 and 1
argacos3_3=(norm_p31_3^2-a(1,2)^2-a(1,3)^2)/(2*a(1,2)*a(1,3)); %bound acos argument between -1 and 1
argacos3_4=(norm_p31_4^2-a(1,2)^2-a(1,3)^2)/(2*a(1,2)*a(1,3)); %bound acos argument between -1 and 1

Theta_31=acos(max(min(argacos3_1,1),-1));
Theta_32=-acos(max(min(argacos3_1,1),-1));
Theta_33=acos(max(min(argacos3_2,1),-1));
Theta_34=-acos(max(min(argacos3_2,1),-1));
Theta_35=acos(max(min(argacos3_3,1),-1));
Theta_36=-acos(max(min(argacos3_3,1),-1));
Theta_37=acos(max(min(argacos3_4,1),-1));
Theta_38=-acos(max(min(argacos3_4,1),-1));

Theta_21=-atan2(p31_1(2,1),-p31_1(1,1))+asin((a(1,3)*sin(Theta_31))/norm_p31_1);
Theta_22=-atan2(p31_1(2,1),-p31_1(1,1))+asin((a(1,3)*sin(Theta_32))/norm_p31_1);
Theta_23=-atan2(p31_2(2,1),-p31_2(1,1))+asin((a(1,3)*sin(Theta_33))/norm_p31_2);
Theta_24=-atan2(p31_2(2,1),-p31_2(1,1))+asin((a(1,3)*sin(Theta_34))/norm_p31_2);
Theta_25=-atan2(p31_3(2,1),-p31_3(1,1))+asin((a(1,3)*sin(Theta_35))/norm_p31_3);
Theta_26=-atan2(p31_3(2,1),-p31_3(1,1))+asin((a(1,3)*sin(Theta_36))/norm_p31_3);
Theta_27=-atan2(p31_4(2,1),-p31_4(1,1))+asin((a(1,3)*sin(Theta_37))/norm_p31_4);
Theta_28=-atan2(p31_4(2,1),-p31_4(1,1))+asin((a(1,3)*sin(Theta_38))/norm_p31_4);

T21_1=[cos(Theta_21) -sin(Theta_21)*cos(alpha(1,2)) sin(Theta_21)*sin(alpha(1,2)) a(1,2)*cos(Theta_21);
    sin(Theta_21) cos(Theta_21)*cos(alpha(1,2)) -cos(Theta_21)*sin(alpha(1,2)) a(1,2)*sin(Theta_21);
    0 sin(alpha(1,2)) cos(alpha(1,2)) d(1,2);
    0 0 0 1];
T21_2=[cos(Theta_22) -sin(Theta_22)*cos(alpha(1,2)) sin(Theta_22)*sin(alpha(1,2)) a(1,2)*cos(Theta_22);
    sin(Theta_22) cos(Theta_22)*cos(alpha(1,2)) -cos(Theta_22)*sin(alpha(1,2)) a(1,2)*sin(Theta_22);
    0 sin(alpha(1,2)) cos(alpha(1,2)) d(1,2);
    0 0 0 1];
T21_3=[cos(Theta_23) -sin(Theta_23)*cos(alpha(1,2)) sin(Theta_23)*sin(alpha(1,2)) a(1,2)*cos(Theta_23);
    sin(Theta_23) cos(Theta_23)*cos(alpha(1,2)) -cos(Theta_23)*sin(alpha(1,2)) a(1,2)*sin(Theta_23);
    0 sin(alpha(1,2)) cos(alpha(1,2)) d(1,2);
    0 0 0 1];
T21_4=[cos(Theta_24) -sin(Theta_24)*cos(alpha(1,2)) sin(Theta_24)*sin(alpha(1,2)) a(1,2)*cos(Theta_24);
    sin(Theta_24) cos(Theta_24)*cos(alpha(1,2)) -cos(Theta_24)*sin(alpha(1,2)) a(1,2)*sin(Theta_24);
    0 sin(alpha(1,2)) cos(alpha(1,2)) d(1,2);
    0 0 0 1];
T21_5=[cos(Theta_25) -sin(Theta_25)*cos(alpha(1,2)) sin(Theta_25)*sin(alpha(1,2)) a(1,2)*cos(Theta_25);
    sin(Theta_25) cos(Theta_25)*cos(alpha(1,2)) -cos(Theta_25)*sin(alpha(1,2)) a(1,2)*sin(Theta_25);
    0 sin(alpha(1,2)) cos(alpha(1,2)) d(1,2);
    0 0 0 1];
T21_6=[cos(Theta_26) -sin(Theta_26)*cos(alpha(1,2)) sin(Theta_26)*sin(alpha(1,2)) a(1,2)*cos(Theta_26);
    sin(Theta_26) cos(Theta_26)*cos(alpha(1,2)) -cos(Theta_26)*sin(alpha(1,2)) a(1,2)*sin(Theta_26);
    0 sin(alpha(1,2)) cos(alpha(1,2)) d(1,2);
    0 0 0 1];
T21_7=[cos(Theta_27) -sin(Theta_27)*cos(alpha(1,2)) sin(Theta_27)*sin(alpha(1,2)) a(1,2)*cos(Theta_27);
    sin(Theta_27) cos(Theta_27)*cos(alpha(1,2)) -cos(Theta_27)*sin(alpha(1,2)) a(1,2)*sin(Theta_27);
    0 sin(alpha(1,2)) cos(alpha(1,2)) d(1,2);
    0 0 0 1];
T21_8=[cos(Theta_28) -sin(Theta_28)*cos(alpha(1,2)) sin(Theta_28)*sin(alpha(1,2)) a(1,2)*cos(Theta_28);
    sin(Theta_28) cos(Theta_28)*cos(alpha(1,2)) -cos(Theta_28)*sin(alpha(1,2)) a(1,2)*sin(Theta_28);
    0 sin(alpha(1,2)) cos(alpha(1,2)) d(1,2);
    0 0 0 1];



T32_1=[cos(Theta_31) -sin(Theta_31)*cos(alpha(1,3)) sin(Theta_31)*sin(alpha(1,3)) a(1,3)*cos(Theta_31);
    sin(Theta_31) cos(Theta_31)*cos(alpha(1,3)) -cos(Theta_31)*sin(alpha(1,3)) a(1,3)*sin(Theta_31);
    0 sin(alpha(1,3)) cos(alpha(1,3)) d(1,3);
    0 0 0 1];
T32_2=[cos(Theta_32) -sin(Theta_32)*cos(alpha(1,3)) sin(Theta_32)*sin(alpha(1,3)) a(1,3)*cos(Theta_32);
    sin(Theta_32) cos(Theta_32)*cos(alpha(1,3)) -cos(Theta_32)*sin(alpha(1,3)) a(1,3)*sin(Theta_32);
    0 sin(alpha(1,3)) cos(alpha(1,3)) d(1,3);
    0 0 0 1];
T32_3=[cos(Theta_33) -sin(Theta_33)*cos(alpha(1,3)) sin(Theta_33)*sin(alpha(1,3)) a(1,3)*cos(Theta_33);
    sin(Theta_33) cos(Theta_33)*cos(alpha(1,3)) -cos(Theta_33)*sin(alpha(1,3)) a(1,3)*sin(Theta_33);
    0 sin(alpha(1,3)) cos(alpha(1,3)) d(1,3);
    0 0 0 1];
T32_4=[cos(Theta_34) -sin(Theta_34)*cos(alpha(1,3)) sin(Theta_34)*sin(alpha(1,3)) a(1,3)*cos(Theta_34);
    sin(Theta_34) cos(Theta_34)*cos(alpha(1,3)) -cos(Theta_34)*sin(alpha(1,3)) a(1,3)*sin(Theta_34);
    0 sin(alpha(1,3)) cos(alpha(1,3)) d(1,3);
    0 0 0 1];
T32_5=[cos(Theta_35) -sin(Theta_35)*cos(alpha(1,3)) sin(Theta_35)*sin(alpha(1,3)) a(1,3)*cos(Theta_35);
    sin(Theta_35) cos(Theta_35)*cos(alpha(1,3)) -cos(Theta_35)*sin(alpha(1,3)) a(1,3)*sin(Theta_35);
    0 sin(alpha(1,3)) cos(alpha(1,3)) d(1,3);
    0 0 0 1];
T32_6=[cos(Theta_36) -sin(Theta_36)*cos(alpha(1,3)) sin(Theta_36)*sin(alpha(1,3)) a(1,3)*cos(Theta_36);
    sin(Theta_36) cos(Theta_36)*cos(alpha(1,3)) -cos(Theta_36)*sin(alpha(1,3)) a(1,3)*sin(Theta_36);
    0 sin(alpha(1,3)) cos(alpha(1,3)) d(1,3);
    0 0 0 1];
T32_7=[cos(Theta_37) -sin(Theta_37)*cos(alpha(1,3)) sin(Theta_37)*sin(alpha(1,3)) a(1,3)*cos(Theta_37);
    sin(Theta_37) cos(Theta_37)*cos(alpha(1,3)) -cos(Theta_37)*sin(alpha(1,3)) a(1,3)*sin(Theta_37);
    0 sin(alpha(1,3)) cos(alpha(1,3)) d(1,3);
    0 0 0 1];
T32_8=[cos(Theta_38) -sin(Theta_38)*cos(alpha(1,3)) sin(Theta_38)*sin(alpha(1,3)) a(1,3)*cos(Theta_38);
    sin(Theta_38) cos(Theta_38)*cos(alpha(1,3)) -cos(Theta_38)*sin(alpha(1,3)) a(1,3)*sin(Theta_38);
    0 sin(alpha(1,3)) cos(alpha(1,3)) d(1,3);
    0 0 0 1];


T43_1=inv(T21_1*T32_1)*T41_1;
T43_2=inv(T21_2*T32_2)*T41_1;
T43_3=inv(T21_3*T32_3)*T41_2;
T43_4=inv(T21_4*T32_4)*T41_2;
T43_5=inv(T21_5*T32_5)*T41_3;
T43_6=inv(T21_6*T32_6)*T41_3;
T43_7=inv(T21_7*T32_7)*T41_4;
T43_8=inv(T21_8*T32_8)*T41_4;


Theta_41=atan2(T43_1(2,1),T43_1(1,1));
Theta_42=atan2(T43_2(2,1),T43_2(1,1));
Theta_43=atan2(T43_3(2,1),T43_3(1,1));
Theta_44=atan2(T43_4(2,1),T43_4(1,1));
Theta_45=atan2(T43_5(2,1),T43_5(1,1));
Theta_46=atan2(T43_6(2,1),T43_6(1,1));
Theta_47=atan2(T43_7(2,1),T43_7(1,1));
Theta_48=atan2(T43_8(2,1),T43_8(1,1));

Solutions = [Theta_11 Theta_21 Theta_31 Theta_41 Theta_51 Theta_61;
    Theta_11 Theta_22 Theta_32 Theta_42 Theta_51 Theta_61;
    Theta_11 Theta_23 Theta_33 Theta_43 Theta_52 Theta_62;
    Theta_11 Theta_24 Theta_34 Theta_44 Theta_52 Theta_62;
    Theta_12 Theta_25 Theta_35 Theta_45 Theta_53 Theta_63;
    Theta_12 Theta_26 Theta_36 Theta_46 Theta_53 Theta_63;
    Theta_12 Theta_27 Theta_37 Theta_47 Theta_54 Theta_64;
    Theta_12 Theta_28 Theta_38 Theta_48 Theta_54 Theta_64];

error = zeros(8,1);
for i=1:8
    error(i)=norm(q_pre'-Solutions(i,:));
end
[~, index] = min(error);

qd = Solutions(index,:)';

end
